simulink model "while_iterator_subsystem"  (R2017b)
settings: Solver=VariableStepAuto  StartTime=0.0  StopTime=10.0  RelTol=1e-3
settings Model: PauseTimes=0  Creator=ppolcz  LastModifiedBy=ppolcz

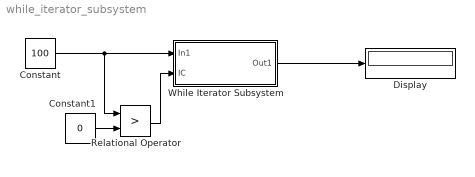
== system while_iterator_subsystem ==
  Constant : Constant  Value=100
  Constant1 : Constant  Value=0
  Display : Display
  Relational Operator : RelationalOperator  Operator=>  OutDataTypeStr=boolean  RndMeth=Nearest
  While Iterator Subsystem : Subsystem  TreatAsAtomicUnit=on
  wires:
  While Iterator Subsystem/1(Out1) -> Display/1
  Constant1/1 -> Relational Operator/2
  Constant/1 -> While Iterator Subsystem/1(In1), Relational Operator/1
  Relational Operator/1 -> While Iterator Subsystem/2(IC)

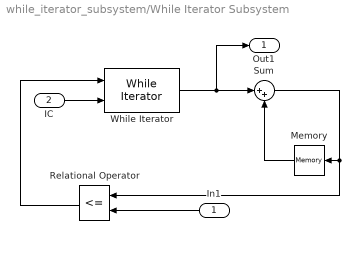
== system while_iterator_subsystem/While Iterator Subsystem ==
  In1 : Inport
  IC : Inport  Port=2
  Memory : Memory  InheritSampleTime=on
  Relational Operator : RelationalOperator  Operator=<=  OutDataTypeStr=boolean  RndMeth=Simplest
  Sum : Sum  Inputs=|++
  While Iterator : WhileIterator  MaxIters=1000  ResetStates=reset  ShowIterationPort=on
  Out1 : Outport
  wires:
  IC/1 -> While Iterator/2
  While Iterator/1 -> Sum/1, Out1/1
  Relational Operator/1 -> While Iterator/1
  Memory/1 -> Sum/2
  Sum/1 -> Relational Operator/1, Memory/1
  In1/1 -> Relational Operator/2
